simulink model "sim_air"  (R2024a)
settings: Solver=VariableStepAuto  StartTime=0.0  StopTime=1000  RelTol=1e-3
values from neighbouring files (symbols this model uses):
  air_temp = params("air_temp")    [eval_air_estimation.m]    (also in eval_noair_estimation.m; gen_data.m)
undefined symbols (not defined in the file or in its folder): current, nominal_soc, oc_voltage, q_gen, sf_temp, terminal_voltage, true_soc, usable_cap
libraries: fl_lib x1, nesl_utility x1
settings Model: DataDictionary=battery.sldd  Creator=Cristobal  LastModifiedBy=n0ne
settings ModelReferenceCC: EnableRefExpFcnMdlSchedulingChecks=on
settings SFSimCC: SimTargetLang=C++  GPUAcceleration=on  SimDLTargetLibrary=cudnn
settings RTWCC: GPUComputeCapability=3.5

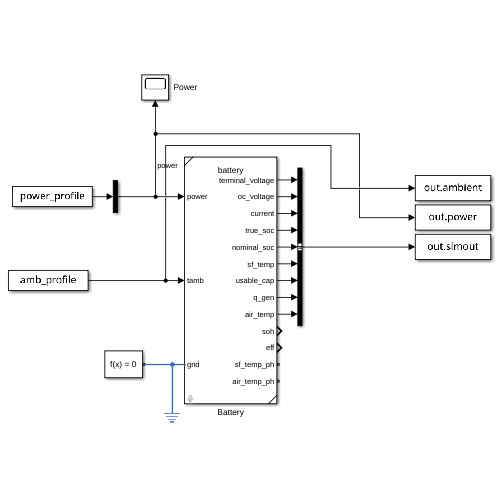
[thumbnail: Simulink's stored preview of the top-level diagram]
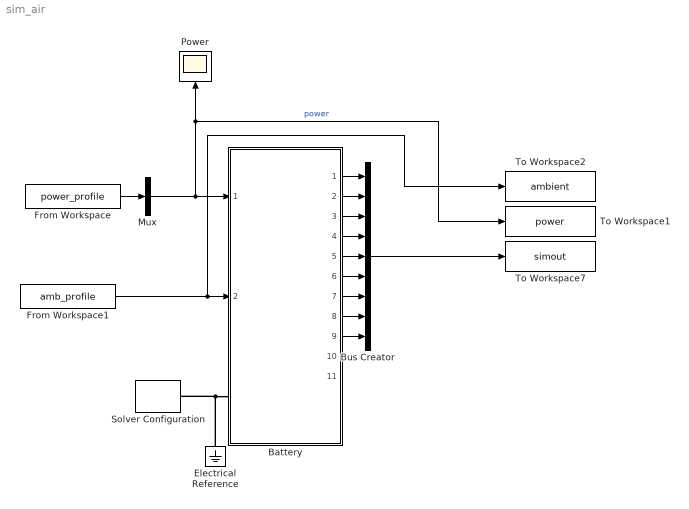
== system sim_air ==
  Battery : Subsystem  ReferencedSubsystem=battery  initial_in_temp=298  initial_air_temp=298  initial_soc=1  initial_soh=1  t_alpha=ALPHA  t_beta=BETA  t_tref=T_REF  ocv_v0=OCV_V0  ocv_vl=OCV_VL  ocv_alpha=OCV_ALPHA  ocv_beta=OCV_BETA  ocv_gamma=OCV_GAMMA  ehc_a=EHC_A  ehc_b=EHC_B  ehc_kappa=EHC_KAPPA  ehc_mu=EHC_MU  ehc_sigma=EHC_SIGMA  ehc_lambda=EHC_LAMBDA  th_cp=HEAT_CAPACITY  th_cair=C_AIR  th_rin=R_IN  th_rout=R_OUT  th_rair=R_AIR
  Bus Creator : BusCreator  Inputs=terminal_voltage,oc_voltage,current,true_soc,nominal_soc,sf_temp,usable_cap,q_gen,air_temp
  Electrical Reference : fl_lib/Electrical/Electrical Elements/Electrical Reference
  From Workspace : FromWorkspace  VariableName=power_profile
  From Workspace1 : FromWorkspace  VariableName=amb_profile
  Mux : Mux  Inputs=1
  Power : Scope
  Solver Configuration : nesl_utility/Solver Configuration  PhysicalDomain=network_engine_domain  SubClassName=solver  LeftPortType=input  RightPortType=generic  Tones=[]  Harmonics=[]  SimulateNoise=off  Profile=off  UseLocalSampling=off  EnableSwitchedLinearOptims=on  FrequencyDomain=off  UseCCode=off  RelTol=0.001  AbsTol=0.001  MinStep=1e-09  ToWorkspace=off  RevertToSquareIcSolve=off  NumHomotopyIterations=100  PhasorMode=off  PhasorModeNumHarmonics=1  ConsistencySolver=NEWTON_FTOL  IndexReductionMethod=DerivativeReplacement  DoDC=off  ResidualTolerance=1e-09  ConsistencyTolSource=GLOBAL  ConsistencyAbsTol=0.001  ConsistencyRelTol=0.001  ConsistencyTolFactor=0.001  UseLocalSolver=off  LocalSolverChoice=NE_BACKWARD_EULER_ADVANCER  ResolveIndetEquations=on  FunctionEvalNumThread=1  LocalSolverSampleTime=0.001  DoFixedCost=off  MaxNonlinIter=3  MaxModeIter=2  ComputeImpulses=off  ImpulseIterations=2  LinearAlgebra=auto  LinearAlgebraNumThread=0  EquationFormulation=NE_TIME_EF  DelaysMemoryBudget=1024  AutomaticFiltering=on  FilteringTimeConstant=0.001  PartitionStorageMethod=AS_NEEDED  PartitionMemoryBudget=1024  PartitionMethod=ROBUST  MultibodyUseLocalSolver=off  MultibodyLocalSolverChoice=ODE1  MultibodyLocalSolverSampleTime=0.001
  To Workspace1 : ToWorkspace  VariableName=power  SaveFormat=Timeseries  SampleTime=-1
  To Workspace2 : ToWorkspace  VariableName=ambient  SaveFormat=Timeseries  SampleTime=-1
  To Workspace7 : ToWorkspace  VariableName=simout  SaveFormat=Timeseries  SampleTime=-1
  wires:
  Bus Creator/1 -> To Workspace7/1
  Battery/3 -> Bus Creator/3
  Battery/4 -> Bus Creator/4
  Battery/5 -> Bus Creator/5
  Battery/6 -> Bus Creator/6
  Battery/7 -> Bus Creator/7
  Battery/1 -> Bus Creator/1
  Battery/2 -> Bus Creator/2
  Battery/8 -> Bus Creator/8
  Mux/1 -> Battery/1, Power/1, To Workspace1/1  "power"
  Battery/9 -> Bus Creator/9
  From Workspace1/1 -> To Workspace2/1, Battery/2
  From Workspace/1 -> Mux/1
  connections:
  Electrical Reference/LConn1 -- Solver Configuration/RConn1 -- Battery/LConn1
